simulink model "ques2"  (R2020b)
settings: Solver=FixedStepAuto  StartTime=0.0  StopTime=5  FixedStep=1/44100  RelTol=1e-3
undefined symbols (not defined in the file or in its folder): DiscIntNeverNeededParam
settings Model: Creator=i7  LastModifiedBy=Alessio

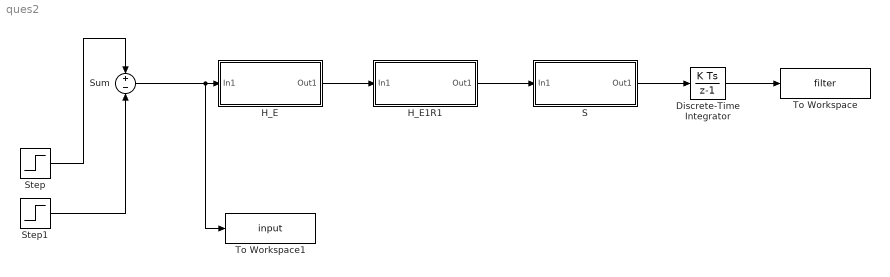
== system ques2 ==
  Discrete-Time Integrator : DiscreteIntegrator  SampleTime=-1  ICPrevOutput=DiscIntNeverNeededParam  ICPrevScaledInput=DiscIntNeverNeededParam
  H_E : Subsystem
  H_E1R1 : Subsystem
  S : Subsystem
  Step : Step  Time=0  SampleTime=0
  Step1 : Step  Time=1/44100  SampleTime=0
  Sum : Sum  Inputs=+-
  To Workspace : ToWorkspace  VariableName=filter  SaveFormat=Timeseries  SampleTime=-1
  To Workspace1 : ToWorkspace  VariableName=input  SaveFormat=Timeseries  SampleTime=-1
  wires:
  H_E/1(Out1) -> H_E1R1/1(In1)
  H_E1R1/1(Out1) -> S/1(In1)
  Step/1 -> Sum/1
  Step1/1 -> Sum/2
  Sum/1 -> To Workspace1/1, H_E/1(In1)
  Discrete-Time Integrator/1 -> To Workspace/1
  S/1(Out1) -> Discrete-Time Integrator/1

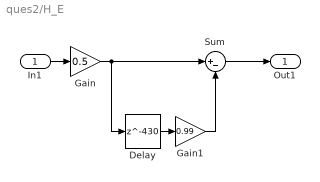
== system ques2/H_E ==
  In1 : Inport
  Delay : Delay  DelayLength=430  InitialCondition=0
  Gain : Gain  Gain=0.5
  Gain1 : Gain  Gain=0.99
  Sum : Sum  Inputs=|+-
  Out1 : Outport
  wires:
  In1/1 -> Gain/1
  Gain/1 -> Delay/1, Sum/1
  Delay/1 -> Gain1/1
  Gain1/1 -> Sum/2
  Sum/1 -> Out1/1

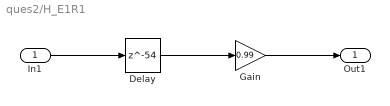
== system ques2/H_E1R1 ==
  In1 : Inport
  Delay : Delay  DelayLength=54  InitialCondition=0
  Gain : Gain  Gain=0.99
  Out1 : Outport
  wires:
  In1/1 -> Delay/1
  Delay/1 -> Gain/1
  Gain/1 -> Out1/1

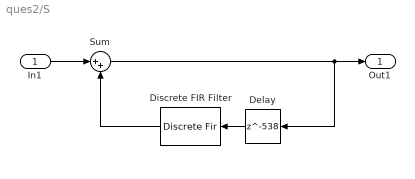
== system ques2/S ==
  In1 : Inport
  Delay : Delay  DelayLength=538  InitialCondition=0
  Discrete FIR Filter : DiscreteFir
  Sum : Sum  Inputs=|++
  Out1 : Outport
  wires:
  In1/1 -> Sum/1
  Sum/1 -> Delay/1, Out1/1
  Delay/1 -> Discrete FIR Filter/1
  Discrete FIR Filter/1 -> Sum/2
